simulink model "lookup_nD_TestGen12"  (R2017b)
settings: Solver=FixedStepDiscrete  StartTime=0.0  StopTime=10.0  RelTol=1e-3
model workspace (MAT data in the model file):
  LUTObjLKnD12 = Simulink.LookupTable
  LUTObjLKnD12.Table = Simulink.lookuptable.Table
  LUTObjLKnD12.Table.Value = [93.5588675269  49.8258659243  73.4080247632  50.3629298657  91.3116756304; 74.4380324496  112.541927759  41.2415969962  92.7327939339  31.8764313321; 92.2905635478  121.954352385  5.36512384972  77.0854583888  6.77392954486]
  LUTObjLKnD12.Table.Dimensions = [3 5]
  LUTObjLKnD12.Table.DataType = 'auto'
  LUTObjLKnD12.Table.FieldName = 'Table'
  LUTObjLKnD12.BreakpointsSpecification = 'Even spacing'
  LUTObjLKnD12.Breakpoints(1) = Simulink.lookuptable.Evenspacing
  LUTObjLKnD12.Breakpoints(1).FirstPoint = 96.3999598398
  LUTObjLKnD12.Breakpoints(1).Spacing = 1.5
  LUTObjLKnD12.Breakpoints(1).FirstPointName = 'BPFirstPoint1'
  LUTObjLKnD12.Breakpoints(1).SpacingName = 'BPSpacing1'
  LUTObjLKnD12.Breakpoints(1).TunableSizeName = 'N1'
  LUTObjLKnD12.Breakpoints(1).DataType = 'auto'
  LUTObjLKnD12.Breakpoints(1).FieldName = 'BP1'
  LUTObjLKnD12.Breakpoints(2) = Simulink.lookuptable.Evenspacing
  LUTObjLKnD12.Breakpoints(2).FirstPoint = 99.8133036157
  LUTObjLKnD12.Breakpoints(2).Spacing = 1.5
  LUTObjLKnD12.Breakpoints(2).FirstPointName = 'BPFirstPoint2'
  LUTObjLKnD12.Breakpoints(2).SpacingName = 'BPSpacing2'
  LUTObjLKnD12.Breakpoints(2).TunableSizeName = 'N2'
  LUTObjLKnD12.Breakpoints(2).DataType = 'auto'
  LUTObjLKnD12.Breakpoints(2).FieldName = 'BP2'
  LUTObjLKnD12.SupportTunableSize = 0
  LUTObjLKnD12.StructTypeInfo = Simulink.lookuptable.StructTypeInfo
  LUTObjLKnD12.StructTypeInfo.Name = 'LUT'
  LUTObjLKnD12.StructTypeInfo.DataScope = 'Auto'
settings Model: Creator=ktrinh  LastModifiedBy=ktrinh
settings DebuggingCC: ParameterOverflowMsg=none

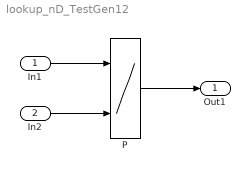
== system lookup_nD_TestGen12 ==
  In1 : Inport  OutMin=0  OutMax=127  PortDimensions=3
  In2 : Inport  Port=2  OutMin=0  OutMax=127
  P : Lookup_n-D  DataSpecification=Lookup table object  LookupTableObject=LUTObjLKnD12  BreakpointsSpecification=Even spacing  BreakpointsForDimension3=[5, 7]  Table=reshape(repmat([4 5 6;16 19 20;10 18 23],1,2),[3,3,2])  UseLastTableValue=on  InternalRulePriority=Speed  RndMeth=Simplest  InputSameDT=on
  Out1 : Outport
  wires:
  In1/1 -> P/1
  In2/1 -> P/2
  P/1 -> Out1/1
